simulink library "uavsimBlockset_LiftCoefficientWithStall"  (Simulink 8.0)
settings: Solver=ode45  StartTime=0.0  StopTime=10.0  RelTol=1e-3
settings Model: Creator=mstolle  LastModifiedBy=j.bolting

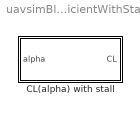
== system uavsimBlockset_LiftCoefficientWithStall ==
  CL(alpha) with stall : Subsystem  mask{mask_M=0, mask_alpha0=0, mask_CL_0=0, mask_CL_alpha=0}
      mask prompts: mask_M "M"; mask_alpha0 "alpha_0"; mask_CL_0 "CL_0"; mask_CL_alpha "CL_alpha"

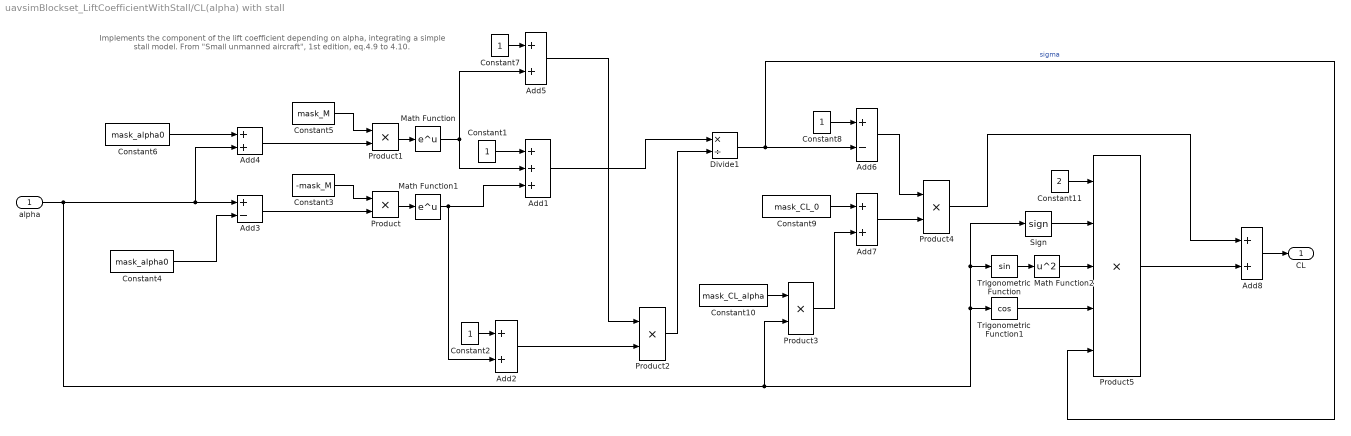
== system uavsimBlockset_LiftCoefficientWithStall/CL(alpha) with stall ==
  note: Implements the component of the lift coefficient depending on alpha,
      | integrating a simple stall model. From "Small unmanned aircraft", 1st edition,  eq.4.9 to 4.10.
  alpha : Inport
  Add1 : Sum  Inputs=+++
  Add{2,4..5,7..8} (5 alike) : Sum
  Add3 : Sum  Inputs=+-
  Add6 : Sum  Inputs=+-
  Constant{1..2,7..8} (4 alike) : Constant
  Constant10 : Constant  Value=mask_CL_alpha
  Constant11 : Constant  Value=2
  Constant3 : Constant  Value=-mask_M
  Constant4 : Constant  Value=mask_alpha0
  Constant5 : Constant  Value=mask_M
  Constant6 : Constant  Value=mask_alpha0
  Constant9 : Constant  Value=mask_CL_0
  Divide1 : Product  Inputs=*/
  Math Function : Math  SaturateOnIntegerOverflow=on
  Math Function1 : Math  SaturateOnIntegerOverflow=on
  Math Function2 : Math  Operator=square  SaturateOnIntegerOverflow=on
  Product{,1..4} (5 alike) : Product  RndMeth=Zero
  Product5 : Product  Inputs=5  RndMeth=Zero
  Sign : Signum
  Trigonometric Function : Trigonometry
  Trigonometric Function1 : Trigonometry  Operator=cos
  CL : Outport
  wires:
  Constant3/1 -> Product/1
  alpha/1 -> Add4/2, Add3/1, Trigonometric Function1/1, Sign/1, Trigonometric Function/1, Product3/2
  Constant4/1 -> Add3/2
  Add3/1 -> Product/2
  Constant5/1 -> Product1/1
  Constant6/1 -> Add4/1
  Add4/1 -> Product1/2
  Product1/1 -> Math Function/1
  Product/1 -> Math Function1/1
  Constant1/1 -> Add1/1
  Math Function/1 -> Add1/2, Add5/2
  Math Function1/1 -> Add2/2, Add1/3
  Constant2/1 -> Add2/1
  Constant7/1 -> Add5/1
  Add2/1 -> Product2/2
  Add5/1 -> Product2/1
  Add1/1 -> Divide1/1
  Product2/1 -> Divide1/2
  Constant8/1 -> Add6/1
  Divide1/1 -> Product5/5, Add6/2  "sigma"
  Constant9/1 -> Add7/1
  Constant10/1 -> Product3/1
  Product3/1 -> Add7/2
  Add6/1 -> Product4/1
  Add7/1 -> Product4/2
  Constant11/1 -> Product5/1
  Sign/1 -> Product5/2
  Math Function2/1 -> Product5/3
  Trigonometric Function/1 -> Math Function2/1
  Trigonometric Function1/1 -> Product5/4
  Product5/1 -> Add8/2
  Product4/1 -> Add8/1
  Add8/1 -> CL/1
